simulink model "Lab_PMSM"  (R2024a)
settings: Solver=VariableStepAuto  StartTime=0.0  StopTime=10  RelTol=1e-3
libraries: spsabctoAlphaBetaZeroLib x1
settings Model: Creator=VICTUS  LastModifiedBy=VICTUS

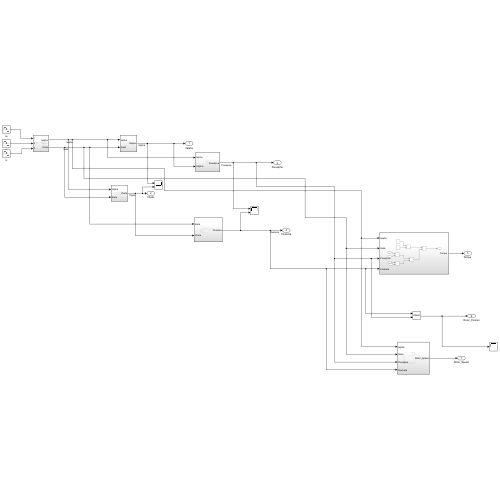
[thumbnail: Simulink's stored preview of the top-level diagram]
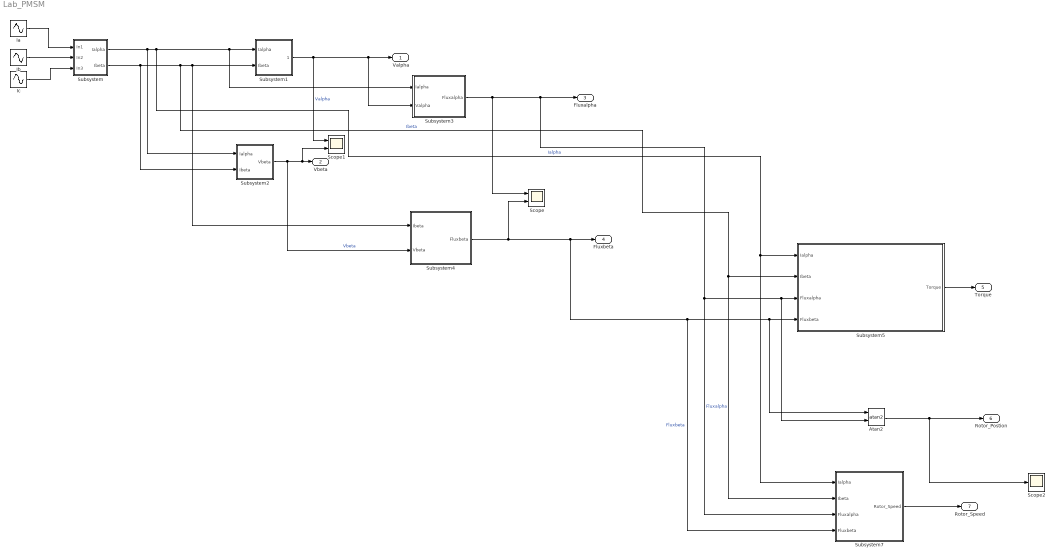
== system Lab_PMSM ==
  Atan2 : Trigonometry  Operator=atan2
  Ia : Sin  Amplitude=2  Frequency=300  SampleTime=0
  Ib : Sin  Amplitude=2  Frequency=300  Phase=-(120/180)*pi  SampleTime=0
  Ic : Sin  Amplitude=2  Frequency=300  Phase=(120/180)*pi  SampleTime=0
  Scope : Scope  NumInputPorts=2
  Scope1 : Scope  NumInputPorts=2
  Scope2 : Scope
  Subsystem : Subsystem
  Subsystem1 : Subsystem
  Subsystem2 : Subsystem
  Subsystem3 : Subsystem
  Subsystem4 : Subsystem
  Subsystem5 : Subsystem
  Subsystem7 : Subsystem
  Valpha : Outport
  Vbeta : Outport  Port=2
  Fluxalpha : Outport  Port=3
  Fluxbeta : Outport  Port=4
  "Torque " : Outport  Port=5
  Rotor_Postion : Outport  Port=6
  Rotor_Speed : Outport  Port=7
  wires:
  Ia/1 -> Subsystem/1(In1)
  Ib/1 -> Subsystem/2(In2)
  Ic/1 -> Subsystem/3(In3)
  Subsystem/1(Ialpha) -> Subsystem2/1(Ialpha), Subsystem7/1(Ialpha), Subsystem5/1(Ialpha), Subsystem3/1(Ialpha), Subsystem1/1(Ialpha)  "Ialpha"
  Subsystem/2(Ibeta) -> Subsystem2/2(Ibeta), Subsystem7/2(Ibeta), Subsystem5/2(Ibeta), Subsystem1/2(Ibeta), Subsystem4/1(Ibeta)  "Ibeta"
  Subsystem1/1(Valpha) -> Scope1/1, Subsystem3/2(Valpha), Valpha/1  "Valpha"
  Subsystem2/1(Vbeta) -> Subsystem4/2(Vbeta), Scope1/2, Vbeta/1  "Vbeta"
  Subsystem3/1(Fluxalpha) -> Scope/1, Subsystem7/3(Fluxalpha), Atan2/2, Subsystem5/3(Fluxalpha), Fluxalpha/1  "Fluxalpha"
  Subsystem4/1(Fluxbeta) -> Scope/2, Subsystem7/4(Fluxbeta), Atan2/1, Subsystem5/4(Fluxbeta), Fluxbeta/1  "Fluxbeta"
  Subsystem5/1("Torque ") -> "Torque "/1
  Subsystem7/1(Rotor_Speed) -> Rotor_Speed/1
  Atan2/1 -> Scope2/1, Rotor_Postion/1

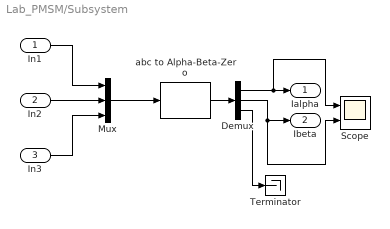
== system Lab_PMSM/Subsystem ==
  In1 : Inport
  In2 : Inport  Port=2
  In3 : Inport  Port=3
  Demux : Demux  Outputs=3
  Mux : Mux  Inputs=3
  Scope : Scope  NumInputPorts=2
  Terminator : Terminator
  abc to Alpha-Beta-Zero : spsabctoAlphaBetaZeroLib/abc to Alpha-Beta-Zero
  Ialpha : Outport
  Ibeta : Outport  Port=2
  wires:
  Mux/1 -> abc to Alpha-Beta-Zero/1
  In1/1 -> Mux/1
  Demux/1 -> Scope/1, Ialpha/1
  abc to Alpha-Beta-Zero/1 -> Demux/1
  Demux/2 -> Scope/2, Ibeta/1
  In2/1 -> Mux/2
  In3/1 -> Mux/3
  Demux/3 -> Terminator/1

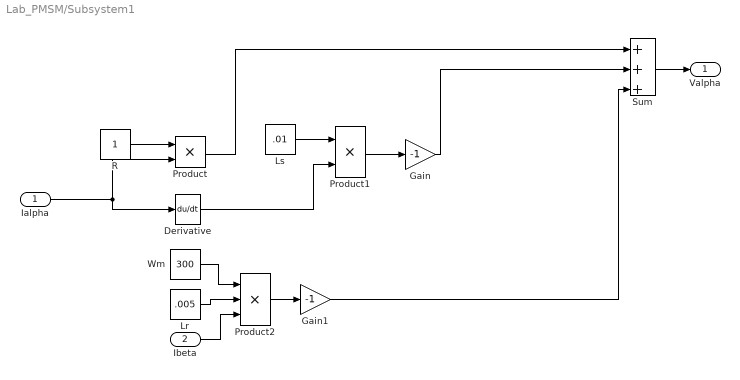
== system Lab_PMSM/Subsystem1 ==
  Ialpha : Inport
  Ibeta : Inport  Port=2
  Derivative : Derivative
  Gain : Gain  Gain=-1
  Gain1 : Gain  Gain=-1
  Lr : Constant  Value=.005
  Ls : Constant  Value=.01
  Product : Product
  Product1 : Product
  Product2 : Product  Inputs=3
  R : Constant
  Sum : Sum  Inputs=|+++
  Wm : Constant  Value=300
  Valpha : Outport
  wires:
  Lr/1 -> Product2/2
  Product2/1 -> Gain1/1
  Wm/1 -> Product2/1
  Product1/1 -> Gain/1
  R/1 -> Product/1
  Gain/1 -> Sum/2
  Ialpha/1 -> Product/2, Derivative/1
  Derivative/1 -> Product1/2
  Product/1 -> Sum/1
  Ls/1 -> Product1/1
  Gain1/1 -> Sum/3
  Ibeta/1 -> Product2/3
  Sum/1 -> Valpha/1

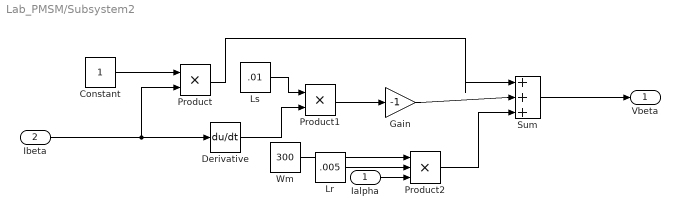
== system Lab_PMSM/Subsystem2 ==
  Ialpha : Inport
  Ibeta : Inport  Port=2
  Constant : Constant
  Derivative : Derivative
  Gain : Gain  Gain=-1
  Lr : Constant  Value=.005
  Ls : Constant  Value=.01
  Product : Product
  Product1 : Product
  Product2 : Product  Inputs=3
  Sum : Sum  Inputs=|+++
  Wm : Constant  Value=300
  Vbeta : Outport
  wires:
  Product/1 -> Sum/1
  Product2/1 -> Sum/3
  Lr/1 -> Product2/2
  Gain/1 -> Sum/2
  Wm/1 -> Product2/1
  Constant/1 -> Product/1
  Ls/1 -> Product1/1
  Derivative/1 -> Product1/2
  Product1/1 -> Gain/1
  Ibeta/1 -> Product/2, Derivative/1
  Ialpha/1 -> Product2/3
  Sum/1 -> Vbeta/1

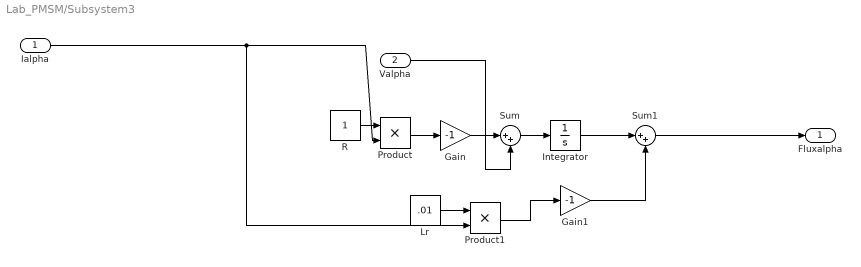
== system Lab_PMSM/Subsystem3 ==
  Ialpha : Inport
  Valpha : Inport  Port=2
  Gain : Gain  Gain=-1
  Gain1 : Gain  Gain=-1
  Integrator : Integrator
  Lr : Constant  Value=.01
  Product : Product
  Product1 : Product
  R : Constant
  Sum : Sum  Inputs=|++
  Sum1 : Sum  Inputs=|++
  Fluxalpha : Outport
  wires:
  Sum/1 -> Integrator/1
  R/1 -> Product/1
  Integrator/1 -> Sum1/1
  Product/1 -> Gain/1
  Product1/1 -> Gain1/1
  Gain1/1 -> Sum1/2
  Lr/1 -> Product1/1
  Gain/1 -> Sum/1
  Ialpha/1 -> Product1/2, Product/2
  Sum1/1 -> Fluxalpha/1
  Valpha/1 -> Sum/2

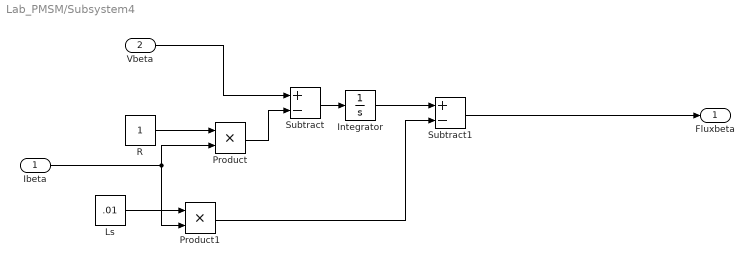
== system Lab_PMSM/Subsystem4 ==
  Ibeta : Inport
  Vbeta : Inport  Port=2
  Integrator : Integrator
  Ls : Constant  Value=.01
  Product : Product
  Product1 : Product
  R : Constant
  Subtract : Sum  Inputs=+-
  Subtract1 : Sum  Inputs=+-
  Fluxbeta : Outport
  wires:
  Subtract/1 -> Integrator/1
  Product1/1 -> Subtract1/2
  Ibeta/1 -> Product/2, Product1/2
  Product/1 -> Subtract/2
  Integrator/1 -> Subtract1/1
  Ls/1 -> Product1/1
  R/1 -> Product/1
  Subtract1/1 -> Fluxbeta/1
  Vbeta/1 -> Subtract/1

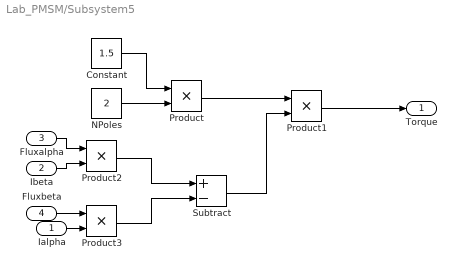
== system Lab_PMSM/Subsystem5 ==
  Ialpha : Inport
  Ibeta : Inport  Port=2
  Fluxalpha : Inport  Port=3
  Fluxbeta : Inport  Port=4
  Constant : Constant  Value=1.5
  NPoles : Constant  Value=2
  Product{,1..3} (4 alike) : Product
  Subtract : Sum  Inputs=+-
  "Torque " : Outport
  wires:
  NPoles/1 -> Product/2
  Subtract/1 -> Product1/2
  Fluxbeta/1 -> Product3/1
  Product/1 -> Product1/1
  Ibeta/1 -> Product2/2
  Product3/1 -> Subtract/2
  Product1/1 -> "Torque "/1
  Product2/1 -> Subtract/1
  Constant/1 -> Product/1
  Ialpha/1 -> Product3/2
  Fluxalpha/1 -> Product2/1

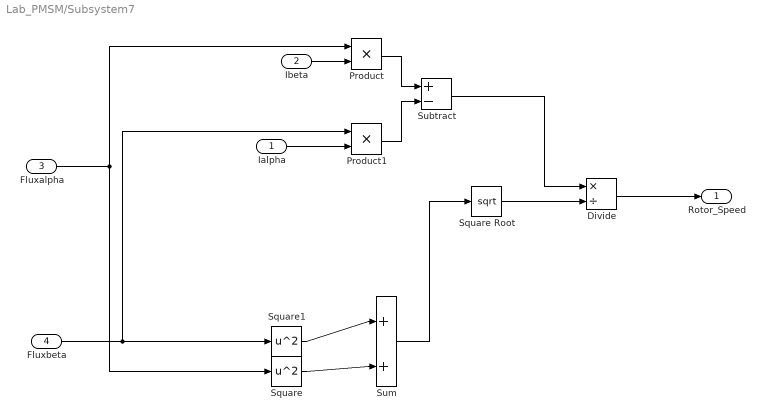
== system Lab_PMSM/Subsystem7 ==
  Ialpha : Inport
  Ibeta : Inport  Port=2
  Fluxalpha : Inport  Port=3
  Fluxbeta : Inport  Port=4
  Divide : Product  Inputs=*/
  Product : Product
  Product1 : Product
  Square : Math  Operator=square
  Square Root : Sqrt
  Square1 : Math  Operator=square
  Subtract : Sum  Inputs=+-
  Sum : Sum  Inputs=|++
  Rotor_Speed : Outport
  wires:
  Product/1 -> Subtract/1
  Square/1 -> Sum/2
  Square1/1 -> Sum/1
  Divide/1 -> Rotor_Speed/1
  Ibeta/1 -> Product/2
  Square Root/1 -> Divide/2
  Subtract/1 -> Divide/1
  Fluxbeta/1 -> Product1/1, Square1/1
  Product1/1 -> Subtract/2
  Sum/1 -> Square Root/1
  Fluxalpha/1 -> Product/1, Square/1
  Ialpha/1 -> Product1/2
